simulink model "mrefrobotarm_previous_y_previous_u_previous_ref_cex"  (R2018b)
settings: Solver=FixedStepAuto  StartTime=0.0  StopTime=20  RelTol=1e-3  AbsTol=1e-6
undefined symbols (not defined in the file or in its folder): cc, options
libraries: neural x330, simulink x2
(part 9 of 13)

== system mrefrobotarm_previous_y_previous_u_previous_ref_cex/cex_m3/Layer 3/Delays 1 ==
  "p{3}" : Inport  PortDimensions=30
      mask Display: e = 0.06;c1 = [120 230 180]/255;c2 = ([120 230 180]+0)/(256+128);c3 = ([120 230 180]+128)/(256+128);patch([0 1 1 0],[0 0 1 1],c1);patch([0 1 1 1-e 1-e 0+e],[0 0 1 1-e 0+e 0+e],c2);patch([0 0 1 1-e 0+e 0+e],[0 1 1 1-e 1-e 0+e],c3);plot([0 1 1 0 0],[0 0 1 1 0]);
  mux : Mux  Inputs=1
      mask Display: e = 0.06;c1 = [120 150 230]/255;c2 = ([120 150 230]+0)/383;c3 = ([120 150 230]+128)/383;patch([0 1 1 0],[0 0 1 1],c1);patch([0 1 1 1-e 1-e 0+e],[0 0 1 1-e 0+e 0+e],c2);patch([0 0 1 1-e 0+e 0+e],[0 1 1 1-e 1-e 0+e],c3);plot([0 1 1 0 0],[0 0 1 1 0]);disp('Mux')
  "pd{3,2}" : Outport
      mask Display: e = 0.06;c1 = [120 230 180]/255;c2 = ([120 230 180]+0)/(256+128);c3 = ([120 230 180]+128)/(256+128);patch([0 1 1 0],[0 0 1 1],c1);patch([0 1 1 1-e 1-e 0+e],[0 0 1 1-e 0+e 0+e],c2);patch([0 0 1 1-e 0+e 0+e],[0 1 1 1-e 1-e 0+e],c3);plot([0 1 1 0 0],[0 0 1 1 0]);
  wires:
  "p{3}"/1 -> mux/1
  mux/1 -> "pd{3,2}"/1

== system mrefrobotarm_previous_y_previous_u_previous_ref_cex/cex_m3/Layer 3/LW{3,2} ==
  "ad{3,2}" : Inport  PortDimensions=30
      mask Display: e = 0.06;c1 = [120 230 180]/255;c2 = ([120 230 180]+0)/(256+128);c3 = ([120 230 180]+128)/(256+128);patch([0 1 1 0],[0 0 1 1],c1);patch([0 1 1 1-e 1-e 0+e],[0 0 1 1-e 0+e 0+e],c2);patch([0 0 1 1-e 0+e 0+e],[0 1 1 1-e 1-e 0+e],c3);plot([0 1 1 0 0],[0 0 1 1 0]);
  "IW{3,2}(1,:)'" : Constant  Value=[-0.4264094248819685351037378495675511658191680908203125;-0.391491550571647362044558349225553683936595916748046875;-0.207148976525499239897953884792514145374298095703125;0.438864475537191156551131143714883364737033843994140625;-0.253842970429255465614204467783565632998943328857421875;-0.310782373552643986780452678431174717843532562255859375;0.17090784249601165267762326038791798055171966552734375;0.48173109431363936305814377192291431128978729248046875;0.282586899793619117371434867891366593539714813232421875;0.01002122853356772480548642079156707040965557098388671875;-0.306381368505943496582943907924345694482326507568359375;0.099394743635973725748300466875662095844745635986328125;-0.320608327918287805413655178199405781924724578857421875;-0.250902128691253001324668048255261965095996856689453125;-0.080231422707110755521142664292710833251476287841796875;0.0929087546576900236150464706952334381639957427978515625;-0.1540763130365487565409665648985537700355052947998046875;0.280406867713617113935242741717956960201263427734375;-0.4379282806221624912978995780576951801776885986328125;0.304633634951007536972866773794521577656269073486328125;-0.09742255331069239743246868101778090931475162506103515625;-0.0928910076785210703231854267869493924081325531005859375;0.475898592804404330092182817679713480174541473388671875;0.0086807129518768309794918280886122374795377254486083984375;-0.479191188062265016611718237982131540775299072265625;0.2631734648013746014072467005462385714054107666015625;-0.010127174248898966613108285628186422400176525115966796875;-0.359889086073808706078835939479176886379718780517578125;-0.01097745989372158649521882267663386301137506961822509765625;-0.12277942593390335501712939958451897837221622467041015625]
      mask Display: e = 0.06;c1 = [120 150 230]/255;c2 = ([120 150 230]+0)/383;c3 = ([120 150 230]+128)/383;patch([0 1 1 0],[0 0 1 1],c1);patch([0 1 1 1-e 1-e 0+e],[0 0 1 1-e 0+e 0+e],c2);patch([0 0 1 1-e 0+e 0+e],[0 1 1 1-e 1-e 0+e],c3);plot([0 1 1 0 0],[0 0 1 1 0]);disp('weights');
  Mux : Mux  Inputs=1
      mask Display: e = 0.06;c1 = [120 150 230]/255;c2 = ([120 150 230]+0)/383;c3 = ([120 150 230]+128)/383;patch([0 1 1 0],[0 0 1 1],c1);patch([0 1 1 1-e 1-e 0+e],[0 0 1 1-e 0+e 0+e],c2);patch([0 0 1 1-e 0+e 0+e],[0 1 1 1-e 1-e 0+e],c3);plot([0 1 1 0 0],[0 0 1 1 0]);disp('Mux');
  dotprod1 : neural/Weight Functions/dotprod
  "lz{3,2}" : Outport
      mask Display: e = 0.06;c1 = [120 230 180]/255;c2 = ([120 230 180]+0)/(256+128);c3 = ([120 230 180]+128)/(256+128);patch([0 1 1 0],[0 0 1 1],c1);patch([0 1 1 1-e 1-e 0+e],[0 0 1 1-e 0+e 0+e],c2);patch([0 0 1 1-e 0+e 0+e],[0 1 1 1-e 1-e 0+e],c3);plot([0 1 1 0 0],[0 0 1 1 0]);
  wires:
  "IW{3,2}(1,:)'"/1 -> dotprod1/1
  "ad{3,2}"/1 -> dotprod1/2
  dotprod1/1 -> Mux/1
  Mux/1 -> "lz{3,2}"/1

== system mrefrobotarm_previous_y_previous_u_previous_ref_cex/cex_m4/Layer 1/Delays 1 ==
  "p{1}" : Inport  PortDimensions=10
      mask Display: e = 0.06;c1 = [120 230 180]/255;c2 = ([120 230 180]+0)/(256+128);c3 = ([120 230 180]+128)/(256+128);patch([0 1 1 0],[0 0 1 1],c1);patch([0 1 1 1-e 1-e 0+e],[0 0 1 1-e 0+e 0+e],c2);patch([0 0 1 1-e 0+e 0+e],[0 1 1 1-e 1-e 0+e],c3);plot([0 1 1 0 0],[0 0 1 1 0]);
  mux : Mux  Inputs=1
      mask Display: e = 0.06;c1 = [120 150 230]/255;c2 = ([120 150 230]+0)/383;c3 = ([120 150 230]+128)/383;patch([0 1 1 0],[0 0 1 1],c1);patch([0 1 1 1-e 1-e 0+e],[0 0 1 1-e 0+e 0+e],c2);patch([0 0 1 1-e 0+e 0+e],[0 1 1 1-e 1-e 0+e],c3);plot([0 1 1 0 0],[0 0 1 1 0]);disp('Mux')
  "pd{1,1}" : Outport
      mask Display: e = 0.06;c1 = [120 230 180]/255;c2 = ([120 230 180]+0)/(256+128);c3 = ([120 230 180]+128)/(256+128);patch([0 1 1 0],[0 0 1 1],c1);patch([0 1 1 1-e 1-e 0+e],[0 0 1 1-e 0+e 0+e],c2);patch([0 0 1 1-e 0+e 0+e],[0 1 1 1-e 1-e 0+e],c3);plot([0 1 1 0 0],[0 0 1 1 0]);
  wires:
  "p{1}"/1 -> mux/1
  mux/1 -> "pd{1,1}"/1

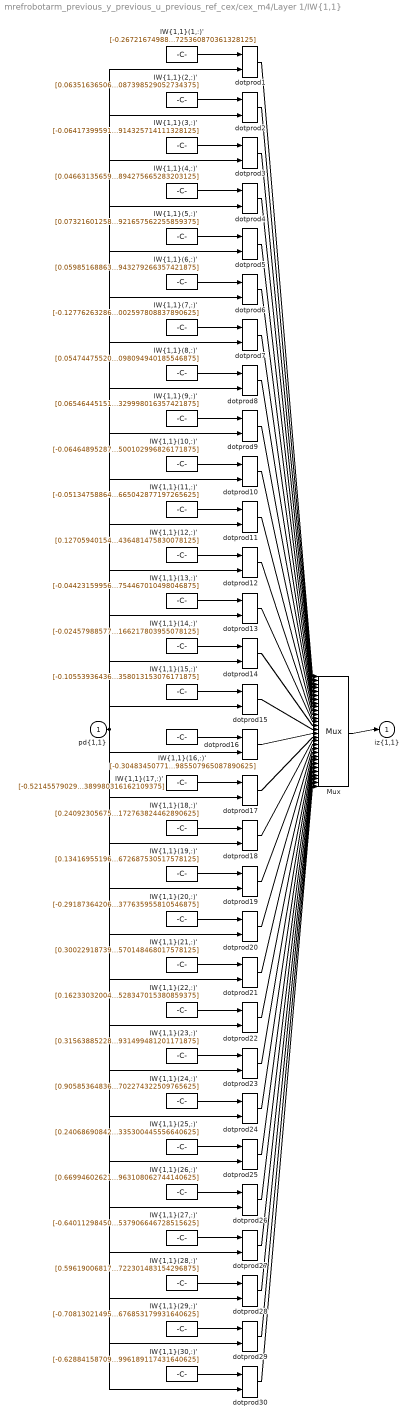
== system mrefrobotarm_previous_y_previous_u_previous_ref_cex/cex_m4/Layer 1/IW{1,1} ==
  "pd{1,1}" : Inport  PortDimensions=10
      mask Display: e = 0.06;c1 = [120 230 180]/255;c2 = ([120 230 180]+0)/(256+128);c3 = ([120 230 180]+128)/(256+128);patch([0 1 1 0],[0 0 1 1],c1);patch([0 1 1 1-e 1-e 0+e],[0 0 1 1-e 0+e 0+e],c2);patch([0 0 1 1-e 0+e 0+e],[0 1 1 1-e 1-e 0+e],c3);plot([0 1 1 0 0],[0 0 1 1 0]);
  "IW{1,1}(1,:)'" : Constant  Value=[-0.267216749881550141854091862114728428423404693603515625;-0.40822662087511296657993398184771649539470672607421875;-0.1379052433439487967969938608803204260766506195068359375;-0.10101957390506945133612504150733002461493015289306640625;-0.218242408285421018998562203705660067498683929443359375;-0.2333909870530341823524622668628580868244171142578125;-0.03607935037657590549020625303455744870007038116455078125;-0.204693462346923371608653496878105215728282928466796875;-0.0676737171591259289993303127630497328937053680419921875;-0.20060575168549832358877438309718854725360870361328125]
      mask Display: e = 0.06;c1 = [120 150 230]/255;c2 = ([120 150 230]+0)/383;c3 = ([120 150 230]+128)/383;patch([0 1 1 0],[0 0 1 1],c1);patch([0 1 1 1-e 1-e 0+e],[0 0 1 1-e 0+e 0+e],c2);patch([0 0 1 1-e 0+e 0+e],[0 1 1 1-e 1-e 0+e],c3);plot([0 1 1 0 0],[0 0 1 1 0]);disp('Weights');
  "IW{1,1}(10,:)'" : Constant  Value=[-0.06464895287319265271275270379192079417407512664794921875;0.0921228152977635883491558388413977809250354766845703125;0.0699758923557921852509622340221540071070194244384765625;0.039369719078938207601492393905573408119380474090576171875;0.2500761972795400023272804901353083550930023193359375;0.1424100538986860231549513855497934855520725250244140625;0.263550719297620916758972953175543807446956634521484375;0.178657006480026581130005070008337497711181640625;0.2561415896215992749063161681988276541233062744140625;-0.06333407118773848321069408484618179500102996826171875]
      mask Display: e = 0.06;c1 = [120 150 230]/255;c2 = ([120 150 230]+0)/383;c3 = ([120 150 230]+128)/383;patch([0 1 1 0],[0 0 1 1],c1);patch([0 1 1 1-e 1-e 0+e],[0 0 1 1-e 0+e 0+e],c2);patch([0 0 1 1-e 0+e 0+e],[0 1 1 1-e 1-e 0+e],c3);plot([0 1 1 0 0],[0 0 1 1 0]);disp('Weights');
  "IW{1,1}(11,:)'" : Constant  Value=[-0.051347588641863818603727764866562210954725742340087890625;0.261299948635366818816549994153319858014583587646484375;-0.07888061835908306840270398652137373574078083038330078125;-0.1396680730473503773136911831898032687604427337646484375;0.07888813015034022713134476134655415080487728118896484375;-0.03396823063257743691156775867057149298489093780517578125;-0.05818663428141730709075574168309685774147510528564453125;-0.207754130607128162377961189122288487851619720458984375;0.121149594677301630785137831480824388563632965087890625;-0.023398605256528072493527048436590121127665042877197265625]
      mask Display: e = 0.06;c1 = [120 150 230]/255;c2 = ([120 150 230]+0)/383;c3 = ([120 150 230]+128)/383;patch([0 1 1 0],[0 0 1 1],c1);patch([0 1 1 1-e 1-e 0+e],[0 0 1 1-e 0+e 0+e],c2);patch([0 0 1 1-e 0+e 0+e],[0 1 1 1-e 1-e 0+e],c3);plot([0 1 1 0 0],[0 0 1 1 0]);disp('Weights');
  "IW{1,1}(12,:)'" : Constant  Value=[0.1270594015435609069886169208984938450157642364501953125;-0.251472209491675646741981609011418186128139495849609375;0.00758860479230148536611277876318126800470054149627685546875;-0.07552348662196907425059322349625290371477603912353515625;-0.0189226418484879331527448442784589133225381374359130859375;-0.151454362118226548705735012845252640545368194580078125;0.006932621563510759678250483517558677704073488712310791015625;0.0379065119537769501523172266388428397476673126220703125;-0.12290012424222727938083465915042324922978878021240234375;0.115999064076067803785718979270313866436481475830078125]
      mask Display: e = 0.06;c1 = [120 150 230]/255;c2 = ([120 150 230]+0)/383;c3 = ([120 150 230]+128)/383;patch([0 1 1 0],[0 0 1 1],c1);patch([0 1 1 1-e 1-e 0+e],[0 0 1 1-e 0+e 0+e],c2);patch([0 0 1 1-e 0+e 0+e],[0 1 1 1-e 1-e 0+e],c3);plot([0 1 1 0 0],[0 0 1 1 0]);disp('Weights');
  "IW{1,1}(13,:)'" : Constant  Value=[-0.04423159956968956973977213920079520903527736663818359375;0.159509068566034528657837654463946819305419921875;-0.03746830256489484811677215247982530854642391204833984375;0.1024420286414695901999749594324384815990924835205078125;-0.1568938236393770668808400614580023102462291717529296875;-0.1263234848339660765237368877933477051556110382080078125;0.1373929609666244833210413389679160900413990020751953125;-0.07214503717479010813651285616288078017532825469970703125;0.0119749599667810895098352119703122298233211040496826171875;-0.07465610010787752937044814416367444209754467010498046875]
      mask Display: e = 0.06;c1 = [120 150 230]/255;c2 = ([120 150 230]+0)/383;c3 = ([120 150 230]+128)/383;patch([0 1 1 0],[0 0 1 1],c1);patch([0 1 1 1-e 1-e 0+e],[0 0 1 1-e 0+e 0+e],c2);patch([0 0 1 1-e 0+e 0+e],[0 1 1 1-e 1-e 0+e],c3);plot([0 1 1 0 0],[0 0 1 1 0]);disp('Weights');
  "IW{1,1}(14,:)'" : Constant  Value=[-0.0245798857762479124045018608057944220490753650665283203125;-0.10986830585016539585385686450536013580858707427978515625;-0.2240634718301251215866187749270466156303882598876953125;0.03927848130053805675299116728638182394206523895263671875;-0.1846276662278691083063364430927322246134281158447265625;0.0260786579550576179398202469883472076617181301116943359375;-0.0923985156179212285820767647237516939640045166015625;-0.060646538855653721322713778363322489894926548004150390625;-0.139029928035326488799938715601456351578235626220703125;0.02460306471988822629715087941804085858166217803955078125]
      mask Display: e = 0.06;c1 = [120 150 230]/255;c2 = ([120 150 230]+0)/383;c3 = ([120 150 230]+128)/383;patch([0 1 1 0],[0 0 1 1],c1);patch([0 1 1 1-e 1-e 0+e],[0 0 1 1-e 0+e 0+e],c2);patch([0 0 1 1-e 0+e 0+e],[0 1 1 1-e 1-e 0+e],c3);plot([0 1 1 0 0],[0 0 1 1 0]);disp('Weights');
  "IW{1,1}(15,:)'" : Constant  Value=[-0.105539364364973742294040448541636578738689422607421875;-0.0263920249190662502269955069778006873093545436859130859375;0.017234595038142376532963595536784850992262363433837890625;-0.255393520989991296143983845468028448522090911865234375;-0.035105650970056238857619490545403095893561840057373046875;-0.0163513867441485612197471510853574727661907672882080078125;-0.0295159521559936639800714175407847505994141101837158203125;-0.1673347691651354551822805660776793956756591796875;-0.037162506725512085836715669984187115915119647979736328125;0.005346155951647601871357107228277527610771358013153076171875]
      mask Display: e = 0.06;c1 = [120 150 230]/255;c2 = ([120 150 230]+0)/383;c3 = ([120 150 230]+128)/383;patch([0 1 1 0],[0 0 1 1],c1);patch([0 1 1 1-e 1-e 0+e],[0 0 1 1-e 0+e 0+e],c2);patch([0 0 1 1-e 0+e 0+e],[0 1 1 1-e 1-e 0+e],c3);plot([0 1 1 0 0],[0 0 1 1 0]);disp('Weights');
  "IW{1,1}(16,:)'" : Constant  Value=[-0.30483450771325137917955316879670135676860809326171875;0.056993584964788047975137175171767012216150760650634765625;-0.13938288150145983212979672316578216850757598876953125;-0.0225306251139089745716415080778460833244025707244873046875;0.01359296115692081551029612995762363425455987453460693359375;-0.1309181736384132654915646298832143656909465789794921875;0.09110308662115275402104686008897260762751102447509765625;-0.1684457458518295869254188801278360188007354736328125;-0.04626449882553897163806055914392345584928989410400390625;-0.284806204554836350784086107523762620985507965087890625]
      mask Display: e = 0.06;c1 = [120 150 230]/255;c2 = ([120 150 230]+0)/383;c3 = ([120 150 230]+128)/383;patch([0 1 1 0],[0 0 1 1],c1);patch([0 1 1 1-e 1-e 0+e],[0 0 1 1-e 0+e 0+e],c2);patch([0 0 1 1-e 0+e 0+e],[0 1 1 1-e 1-e 0+e],c3);plot([0 1 1 0 0],[0 0 1 1 0]);disp('Weights');
  "IW{1,1}(17,:)'" : Constant  Value=[-0.52145579029431754491952233365736901760101318359375;-0.324607409752539488589917482386226765811443328857421875;-0.0319440781114496974435468246156233362853527069091796875;-0.01239414051610091514754596886405124678276479244232177734375;-0.1914576463747985346497415548583376221358776092529296875;-0.157309606734231055558126399773755110800266265869140625;-0.32148224800624036756602208697586320340633392333984375;-0.284450749251240420090169891409459523856639862060546875;-0.1478505228260354187330705144631792791187763214111328125;-0.045385020230083082670713423567576683126389980316162109375]
      mask Display: e = 0.06;c1 = [120 150 230]/255;c2 = ([120 150 230]+0)/383;c3 = ([120 150 230]+128)/383;patch([0 1 1 0],[0 0 1 1],c1);patch([0 1 1 1-e 1-e 0+e],[0 0 1 1-e 0+e 0+e],c2);patch([0 0 1 1-e 0+e 0+e],[0 1 1 1-e 1-e 0+e],c3);plot([0 1 1 0 0],[0 0 1 1 0]);disp('Weights');
  "IW{1,1}(18,:)'" : Constant  Value=[0.2409230567548679424749735744626377709209918975830078125;0.49656984646448576459221158074797131121158599853515625;0.290985707265938586818521116583724506199359893798828125;0.352602910642589140177705075984704308211803436279296875;0.3085480397073692149234602766227908432483673095703125;0.222304352434349594691553875236422754824161529541015625;0.303863149672055243843971084061195142567157745361328125;0.0698155688711211419583690940271480940282344818115234375;-0.1600693098387457047326876136139617301523685455322265625;-0.429772611327940590175700208419584669172763824462890625]
      mask Display: e = 0.06;c1 = [120 150 230]/255;c2 = ([120 150 230]+0)/383;c3 = ([120 150 230]+128)/383;patch([0 1 1 0],[0 0 1 1],c1);patch([0 1 1 1-e 1-e 0+e],[0 0 1 1-e 0+e 0+e],c2);patch([0 0 1 1-e 0+e 0+e],[0 1 1 1-e 1-e 0+e],c3);plot([0 1 1 0 0],[0 0 1 1 0]);disp('Weights');
  "IW{1,1}(19,:)'" : Constant  Value=[0.1341695519644230116806937758155982010066509246826171875;-0.1742853076472074269620549102910445071756839752197265625;-0.03701738455975168984313228293103748001158237457275390625;0.076384486426226583244414314322057180106639862060546875;-0.01047937876791799928499759886335596092976629734039306640625;-0.12109423257529740303173326765318051911890506744384765625;0.0220112019456234764280821991633274592459201812744140625;-0.16146623763280143482035100532812066376209259033203125;0.06120155563627853456676319865437108092010021209716796875;-0.08720404259234344757079071541738812811672687530517578125]
      mask Display: e = 0.06;c1 = [120 150 230]/255;c2 = ([120 150 230]+0)/383;c3 = ([120 150 230]+128)/383;patch([0 1 1 0],[0 0 1 1],c1);patch([0 1 1 1-e 1-e 0+e],[0 0 1 1-e 0+e 0+e],c2);patch([0 0 1 1-e 0+e 0+e],[0 1 1 1-e 1-e 0+e],c3);plot([0 1 1 0 0],[0 0 1 1 0]);disp('Weights');
  "IW{1,1}(2,:)'" : Constant  Value=[0.06351636506590928321625000307903974317014217376708984375;0.11930786387308332796575172096709138713777065277099609375;0.1280645820977200644019688979824422858655452728271484375;0.162144232475708138796477442156174220144748687744140625;0.1871883600761256316591385484571219421923160552978515625;0.0168292633844707890944381034614707459695637226104736328125;0.1938829913256168435697901486491900868713855743408203125;0.06509252142771927707176615740536362864077091217041015625;-0.02851669131545607471789338660528301261365413665771484375;-0.318876840320537979778237058781087398529052734375]
      mask Display: e = 0.06;c1 = [120 150 230]/255;c2 = ([120 150 230]+0)/383;c3 = ([120 150 230]+128)/383;patch([0 1 1 0],[0 0 1 1],c1);patch([0 1 1 1-e 1-e 0+e],[0 0 1 1-e 0+e 0+e],c2);patch([0 0 1 1-e 0+e 0+e],[0 1 1 1-e 1-e 0+e],c3);plot([0 1 1 0 0],[0 0 1 1 0]);disp('Weights');
  "IW{1,1}(20,:)'" : Constant  Value=[-0.291873642062524918383559224821510724723339080810546875;0.0155193769184839742980575039155155536718666553497314453125;-0.25462870462001541138619131743325851857662200927734375;-0.046663558636088897646487794190761633217334747314453125;-0.2050390720883230877280567483467166312038898468017578125;-0.2490154875268562328916033266068552620708942413330078125;-0.273116089395899541703016666360781528055667877197265625;-0.289683676595492212157978428876958787441253662109375;-0.132150491808138259575144957125303335487842559814453125;-0.0552559521734092840006269398145377635955810546875]
      mask Display: e = 0.06;c1 = [120 150 230]/255;c2 = ([120 150 230]+0)/383;c3 = ([120 150 230]+128)/383;patch([0 1 1 0],[0 0 1 1],c1);patch([0 1 1 1-e 1-e 0+e],[0 0 1 1-e 0+e 0+e],c2);patch([0 0 1 1-e 0+e 0+e],[0 1 1 1-e 1-e 0+e],c3);plot([0 1 1 0 0],[0 0 1 1 0]);disp('Weights');
  "IW{1,1}(21,:)'" : Constant  Value=[0.300229187392162477632240324965096078813076019287109375;0.317431380612897717785614304375485517084598541259765625;0.11458850033386035194293839367674081586301326751708984375;0.176851946571799256702206548652611672878265380859375;0.07768512346275276148066524228852358646690845489501953125;0.178815523221328043224076509432052262127399444580078125;0.10338050103036089399921593212638981640338897705078125;0.018921033678644443021266141613523359410464763641357421875;0.189488271159305610158440913437516428530216217041015625;0.1903798222345019219847728209060733206570148468017578125]
      mask Display: e = 0.06;c1 = [120 150 230]/255;c2 = ([120 150 230]+0)/383;c3 = ([120 150 230]+128)/383;patch([0 1 1 0],[0 0 1 1],c1);patch([0 1 1 1-e 1-e 0+e],[0 0 1 1-e 0+e 0+e],c2);patch([0 0 1 1-e 0+e 0+e],[0 1 1 1-e 1-e 0+e],c3);plot([0 1 1 0 0],[0 0 1 1 0]);disp('Weights');
  "IW{1,1}(22,:)'" : Constant  Value=[0.162330320040409425974559098904137499630451202392578125;0.1760155520548265795088838103765738196671009063720703125;0.1980011245623203020027602860864135436713695526123046875;0.08825896072960770499804539213073439896106719970703125;0.214221740389516079883236443492933176457881927490234375;0.08709375089588149154717910960243898443877696990966796875;0.1432464034548406595082070680291508324444293975830078125;0.205133408044915255263873632429749704897403717041015625;0.1616554197014331284432131496942020021378993988037109375;0.1410755108505339361357755478820763528347015380859375]
      mask Display: e = 0.06;c1 = [120 150 230]/255;c2 = ([120 150 230]+0)/383;c3 = ([120 150 230]+128)/383;patch([0 1 1 0],[0 0 1 1],c1);patch([0 1 1 1-e 1-e 0+e],[0 0 1 1-e 0+e 0+e],c2);patch([0 0 1 1-e 0+e 0+e],[0 1 1 1-e 1-e 0+e],c3);plot([0 1 1 0 0],[0 0 1 1 0]);disp('Weights');
  "IW{1,1}(23,:)'" : Constant  Value=[0.3156388522827195952658030364545993506908416748046875;-0.0303480675321638748709318633700604550540447235107421875;0.0261651991707960406008393050569793558679521083831787109375;0.052469398667946427761155092639455688185989856719970703125;0.032880744367926283133751752529860823415219783782958984375;0.0942659029548157112454731532125151716172695159912109375;0.142636786970836426657882611834793351590633392333984375;-0.057596112250889619499361060661613009870052337646484375;0.0955492320642383763384941630647517740726470947265625;-0.07794382114178070863896863329500774852931499481201171875]
      mask Display: e = 0.06;c1 = [120 150 230]/255;c2 = ([120 150 230]+0)/383;c3 = ([120 150 230]+128)/383;patch([0 1 1 0],[0 0 1 1],c1);patch([0 1 1 1-e 1-e 0+e],[0 0 1 1-e 0+e 0+e],c2);patch([0 0 1 1-e 0+e 0+e],[0 1 1 1-e 1-e 0+e],c3);plot([0 1 1 0 0],[0 0 1 1 0]);disp('Weights');
  "IW{1,1}(24,:)'" : Constant  Value=[0.90585364836736703697539496715762652456760406494140625;-0.2426328840753690652132235072713228873908519744873046875;0.2290538535864212743575762942782603204250335693359375;0.0276980522269096758603001973142454517073929309844970703125;0.09685979922238562023206753792692325077950954437255859375;0.1261857423448861370562923411853262223303318023681640625;-0.09704113755403249996778214381265570409595966339111328125;0.1577690254322382801266400065287598408758640289306640625;0.025090152047807907920162762138716061599552631378173828125;0.10783235852078067174009134987500146962702274322509765625]
      mask Display: e = 0.06;c1 = [120 150 230]/255;c2 = ([120 150 230]+0)/383;c3 = ([120 150 230]+128)/383;patch([0 1 1 0],[0 0 1 1],c1);patch([0 1 1 1-e 1-e 0+e],[0 0 1 1-e 0+e 0+e],c2);patch([0 0 1 1-e 0+e 0+e],[0 1 1 1-e 1-e 0+e],c3);plot([0 1 1 0 0],[0 0 1 1 0]);disp('Weights');
  "IW{1,1}(25,:)'" : Constant  Value=[0.240686908421116674272610680418438278138637542724609375;-0.104028123549407769399266499021905474364757537841796875;-0.09450604313064690786827526380875497125089168548583984375;0.11409052644208968196881670564835076220333576202392578125;-0.069072497417360823046550422077416442334651947021484375;-0.1277032424560556045367576416538213379681110382080078125;0.060117468374489287097350853628086042590439319610595703125;0.087487371426137716667881250032223761081695556640625;-0.032553856975236307447207906307085067965090274810791015625;0.005567118611491368197763396352684139856137335300445556640625]
      mask Display: e = 0.06;c1 = [120 150 230]/255;c2 = ([120 150 230]+0)/383;c3 = ([120 150 230]+128)/383;patch([0 1 1 0],[0 0 1 1],c1);patch([0 1 1 1-e 1-e 0+e],[0 0 1 1-e 0+e 0+e],c2);patch([0 0 1 1-e 0+e 0+e],[0 1 1 1-e 1-e 0+e],c3);plot([0 1 1 0 0],[0 0 1 1 0]);disp('Weights');
  "IW{1,1}(26,:)'" : Constant  Value=[0.66994602621044474499711895987275056540966033935546875;0.2219850096971208441853917747721425257623195648193359375;0.176049719549269345630904126664972864091396331787109375;0.1226973401518094142215176134413923136889934539794921875;0.07370925043911900897963818124480894766747951507568359375;-0.07340785025997599577696206551991053856909275054931640625;0.042640181004205530979067617636246723122894763946533203125;-0.153863749044390318854169663609354756772518157958984375;-0.04609826544353955168897840621866635046899318695068359375;0.1366000115535325465376814690898754633963108062744140625]
      mask Display: e = 0.06;c1 = [120 150 230]/255;c2 = ([120 150 230]+0)/383;c3 = ([120 150 230]+128)/383;patch([0 1 1 0],[0 0 1 1],c1);patch([0 1 1 1-e 1-e 0+e],[0 0 1 1-e 0+e 0+e],c2);patch([0 0 1 1-e 0+e 0+e],[0 1 1 1-e 1-e 0+e],c3);plot([0 1 1 0 0],[0 0 1 1 0]);disp('Weights');
  "IW{1,1}(27,:)'" : Constant  Value=[-0.64011298450993125985775122899212874472141265869140625;0.1264277862932005336293883601683774031698703765869140625;-0.1885447022138225514620302192270173691213130950927734375;-0.09251043684248581866480520830009481869637966156005859375;0.103092036338989168076096802906249649822711944580078125;-0.00191654901815719908193813569852181899477727711200714111328125;-0.053867495492080121055611385827432968653738498687744140625;-0.039687340519823595397230775461139273829758167266845703125;-0.04914164559390850339770651089565944857895374298095703125;-0.0258128202979643374403995181864956975914537906646728515625]
      mask Display: e = 0.06;c1 = [120 150 230]/255;c2 = ([120 150 230]+0)/383;c3 = ([120 150 230]+128)/383;patch([0 1 1 0],[0 0 1 1],c1);patch([0 1 1 1-e 1-e 0+e],[0 0 1 1-e 0+e 0+e],c2);patch([0 0 1 1-e 0+e 0+e],[0 1 1 1-e 1-e 0+e],c3);plot([0 1 1 0 0],[0 0 1 1 0]);disp('Weights');
  "IW{1,1}(28,:)'" : Constant  Value=[0.5961900681766694187757593681453727185726165771484375;0.3430139714958020391577520058490335941314697265625;0.2341959314177390061306738289204076863825321197509765625;0.239631643975415087322033969030599109828472137451171875;0.1870724775690954799767240501751075498759746551513671875;0.1467603001405427820547089368119486607611179351806640625;0.10365323923488352353405872463554260320961475372314453125;0.1159775255986031095023491843676310963928699493408203125;0.05082354533000295326861106559590552933514118194580078125;-0.276042206131973333338436304984497837722301483154296875]
      mask Display: e = 0.06;c1 = [120 150 230]/255;c2 = ([120 150 230]+0)/383;c3 = ([120 150 230]+128)/383;patch([0 1 1 0],[0 0 1 1],c1);patch([0 1 1 1-e 1-e 0+e],[0 0 1 1-e 0+e 0+e],c2);patch([0 0 1 1-e 0+e 0+e],[0 1 1 1-e 1-e 0+e],c3);plot([0 1 1 0 0],[0 0 1 1 0]);disp('Weights');
  "IW{1,1}(29,:)'" : Constant  Value=[-0.70813021495672179295155501677072606980800628662109375;0.30675665628371129312057519200607202947139739990234375;-0.07076881114415210782819798396303667686879634857177734375;-0.0228481476932857925643549634742157650180160999298095703125;-0.082537316541165306471583562597515992820262908935546875;-0.0173445013735810428523453907700968557037413120269775390625;0.1688513365261939125350210133547079749405384063720703125;-0.07408557471998102050836365606301114894449710845947265625;-0.07749801166984006395299644509577774442732334136962890625;-0.18928142296034311531371940873214043676853179931640625]
      mask Display: e = 0.06;c1 = [120 150 230]/255;c2 = ([120 150 230]+0)/383;c3 = ([120 150 230]+128)/383;patch([0 1 1 0],[0 0 1 1],c1);patch([0 1 1 1-e 1-e 0+e],[0 0 1 1-e 0+e 0+e],c2);patch([0 0 1 1-e 0+e 0+e],[0 1 1 1-e 1-e 0+e],c3);plot([0 1 1 0 0],[0 0 1 1 0]);disp('Weights');
  "IW{1,1}(3,:)'" : Constant  Value=[-0.064173995914235393289715148057439364492893218994140625;-0.0059172667376275987771716557972467853687703609466552734375;0.05749714985246447140898595762337208725512027740478515625;-0.0899378683654476207554040456670918501913547515869140625;0.078819850763461707376933418345288373529911041259765625;0.0253495636063069233745448372019382077269256114959716796875;-0.0182511162189372307118606642006852780468761920928955078125;-0.0924131757659971686535982371424324810504913330078125;0.0010697191710963248334476105583235039375722408294677734375;0.1566136603183161668528811105716158635914325714111328125]
      mask Display: e = 0.06;c1 = [120 150 230]/255;c2 = ([120 150 230]+0)/383;c3 = ([120 150 230]+128)/383;patch([0 1 1 0],[0 0 1 1],c1);patch([0 1 1 1-e 1-e 0+e],[0 0 1 1-e 0+e 0+e],c2);patch([0 0 1 1-e 0+e 0+e],[0 1 1 1-e 1-e 0+e],c3);plot([0 1 1 0 0],[0 0 1 1 0]);disp('Weights');
  "IW{1,1}(30,:)'" : Constant  Value=[-0.628841587095009924013311319868080317974090576171875;0.1088899533473890179902099362152512185275554656982421875;-0.06463334913051617391932524014919181354343891143798828125;-0.043920919679465507401427970535223721526563167572021484375;-0.09722145811493441980299934357390156947076320648193359375;-0.051994330993742461644036012557990034110844135284423828125;0.1151241109324362132948493808726198039948940277099609375;0.0271505797353484117084843063594234990887343883514404296875;-0.0624483511445974859288554625891265459358692169189453125;-0.2341109402932441130307239518515416420996189117431640625]
      mask Display: e = 0.06;c1 = [120 150 230]/255;c2 = ([120 150 230]+0)/383;c3 = ([120 150 230]+128)/383;patch([0 1 1 0],[0 0 1 1],c1);patch([0 1 1 1-e 1-e 0+e],[0 0 1 1-e 0+e 0+e],c2);patch([0 0 1 1-e 0+e 0+e],[0 1 1 1-e 1-e 0+e],c3);plot([0 1 1 0 0],[0 0 1 1 0]);disp('Weights');
  "IW{1,1}(4,:)'" : Constant  Value=[0.0466313565929649398444922780981869436800479888916015625;-0.06226913105247489088611700935871340334415435791015625;-0.01544836403327122346940125652281494694761931896209716796875;0.03466835985496351246748503172057098709046840667724609375;0.07173125569554179847830965854882379062473773956298828125;0.153078658361084196659618328340002335608005523681640625;0.0770878264398895118869603493294562213122844696044921875;0.1874709283106799073692627644049935042858123779296875;0.08115331332375307071824721560915349982678890228271484375;0.0909525515275941831561112849158234894275665283203125]
      mask Display: e = 0.06;c1 = [120 150 230]/255;c2 = ([120 150 230]+0)/383;c3 = ([120 150 230]+128)/383;patch([0 1 1 0],[0 0 1 1],c1);patch([0 1 1 1-e 1-e 0+e],[0 0 1 1-e 0+e 0+e],c2);patch([0 0 1 1-e 0+e 0+e],[0 1 1 1-e 1-e 0+e],c3);plot([0 1 1 0 0],[0 0 1 1 0]);disp('Weights');
  "IW{1,1}(5,:)'" : Constant  Value=[0.07321601258536401812815341827445081435143947601318359375;-0.22569618673739311187631528810015879571437835693359375;0.1376235218885525635190703042098903097212314605712890625;0.0947860079499896757138088787542073987424373626708984375;0.1290056428927640330694970316471881233155727386474609375;0.053390939220054646485724703097730525769293308258056640625;-0.045191743751136388695943679749689181335270404815673828125;0.056231567537908866416529463094775564968585968017578125;-0.2466164700931786357696040568043827079236507415771484375;-0.20638216121557417803700218428275547921657562255859375]
      mask Display: e = 0.06;c1 = [120 150 230]/255;c2 = ([120 150 230]+0)/383;c3 = ([120 150 230]+128)/383;patch([0 1 1 0],[0 0 1 1],c1);patch([0 1 1 1-e 1-e 0+e],[0 0 1 1-e 0+e 0+e],c2);patch([0 0 1 1-e 0+e 0+e],[0 1 1 1-e 1-e 0+e],c3);plot([0 1 1 0 0],[0 0 1 1 0]);disp('Weights');
  "IW{1,1}(6,:)'" : Constant  Value=[0.05985168863605760947166345431469380855560302734375;-0.002159573538259234627700866582244998426176607608795166015625;-0.11318048141550020313506053071250789798796176910400390625;0.045337237095633316219522868095737067051231861114501953125;0.144154365313161336725755745646893046796321868896484375;0.06093673556748956110507009498178376816213130950927734375;-0.060293185465568922831725018340875976718962192535400390625;0.0227417706844570514934655847127942251972854137420654296875;-0.07437535283304806676962783740236773155629634857177734375;0.126522101641080630951563534836168400943279266357421875]
      mask Display: e = 0.06;c1 = [120 150 230]/255;c2 = ([120 150 230]+0)/383;c3 = ([120 150 230]+128)/383;patch([0 1 1 0],[0 0 1 1],c1);patch([0 1 1 1-e 1-e 0+e],[0 0 1 1-e 0+e 0+e],c2);patch([0 0 1 1-e 0+e 0+e],[0 1 1 1-e 1-e 0+e],c3);plot([0 1 1 0 0],[0 0 1 1 0]);disp('Weights');
  "IW{1,1}(7,:)'" : Constant  Value=[-0.1277626328603604921596570420661009848117828369140625;-0.46443151291336259856024071268620900809764862060546875;0.044606677753775601791286220532128936611115932464599609375;-0.136410331273810248031708169946796260774135589599609375;-0.0770422591237390486096359154544188641011714935302734375;-0.051187319207494509643030511369943269528448581695556640625;-0.09003239138660514007117541268598870374262332916259765625;-0.005325811764632123850027323186395733500830829143524169921875;-0.02833124307385037621287438014405779540538787841796875;0.198670566199726617018228580491268076002597808837890625]
      mask Display: e = 0.06;c1 = [120 150 230]/255;c2 = ([120 150 230]+0)/383;c3 = ([120 150 230]+128)/383;patch([0 1 1 0],[0 0 1 1],c1);patch([0 1 1 1-e 1-e 0+e],[0 0 1 1-e 0+e 0+e],c2);patch([0 0 1 1-e 0+e 0+e],[0 1 1 1-e 1-e 0+e],c3);plot([0 1 1 0 0],[0 0 1 1 0]);disp('Weights');
  "IW{1,1}(8,:)'" : Constant  Value=[0.054744755203041874092040330879171960987150669097900390625;-0.001305994968348087904852494745000512921251356601715087890625;-0.09307953323685579094526332255554734729230403900146484375;-0.08109344435434541475959946410512202419340610504150390625;-0.0907065859835935739408085964896599762141704559326171875;-0.0220450076101698366759507052847766317427158355712890625;-0.026212681759366772415997814960064715705811977386474609375;0.1228943021643547073296076632686890661716461181640625;0.08801937892250617789802191737180692143738269805908203125;0.08659338115619912012999037642657640390098094940185546875]
      mask Display: e = 0.06;c1 = [120 150 230]/255;c2 = ([120 150 230]+0)/383;c3 = ([120 150 230]+128)/383;patch([0 1 1 0],[0 0 1 1],c1);patch([0 1 1 1-e 1-e 0+e],[0 0 1 1-e 0+e 0+e],c2);patch([0 0 1 1-e 0+e 0+e],[0 1 1 1-e 1-e 0+e],c3);plot([0 1 1 0 0],[0 0 1 1 0]);disp('Weights');
  "IW{1,1}(9,:)'" : Constant  Value=[0.06546445151039102794410240448996773920953273773193359375;0.38763234071624308452186369322589598596096038818359375;-0.00672576750667506530201311676364639424718916416168212890625;0.110151702288806163654300007692654617130756378173828125;0.1013987501450804573632780147818266414105892181396484375;0.051810761808782891668645476102028624154627323150634765625;0.0494189364730958924365467055395129136741161346435546875;-0.026199443819789280940568687583436258137226104736328125;-0.0025078487207655822226193276236472229356877505779266357421875;-0.279777179941980147503954867715947329998016357421875]
      mask Display: e = 0.06;c1 = [120 150 230]/255;c2 = ([120 150 230]+0)/383;c3 = ([120 150 230]+128)/383;patch([0 1 1 0],[0 0 1 1],c1);patch([0 1 1 1-e 1-e 0+e],[0 0 1 1-e 0+e 0+e],c2);patch([0 0 1 1-e 0+e 0+e],[0 1 1 1-e 1-e 0+e],c3);plot([0 1 1 0 0],[0 0 1 1 0]);disp('Weights');
  Mux : Mux  Inputs=30
      mask Display: e = 0.06;c1 = [120 150 230]/255;c2 = ([120 150 230]+0)/383;c3 = ([120 150 230]+128)/383;patch([0 1 1 0],[0 0 1 1],c1);patch([0 1 1 1-e 1-e 0+e],[0 0 1 1-e 0+e 0+e],c2);patch([0 0 1 1-e 0+e 0+e],[0 1 1 1-e 1-e 0+e],c3);plot([0 1 1 0 0],[0 0 1 1 0]);disp('Mux');
  dotprod{1..30} (30 alike) : neural/Weight Functions/dotprod
  "iz{1,1}" : Outport
      mask Display: e = 0.06;c1 = [120 230 180]/255;c2 = ([120 230 180]+0)/(256+128);c3 = ([120 230 180]+128)/(256+128);patch([0 1 1 0],[0 0 1 1],c1);patch([0 1 1 1-e 1-e 0+e],[0 0 1 1-e 0+e 0+e],c2);patch([0 0 1 1-e 0+e 0+e],[0 1 1 1-e 1-e 0+e],c3);plot([0 1 1 0 0],[0 0 1 1 0]);
  wires:
  "IW{1,1}(1,:)'"/1 -> dotprod1/1
  "pd{1,1}"/1 -> dotprod1/2, dotprod2/2, dotprod3/2, dotprod4/2, dotprod5/2, dotprod6/2, dotprod7/2, dotprod8/2, dotprod9/2, dotprod10/2, dotprod11/2, dotprod12/2, dotprod13/2, dotprod14/2, dotprod15/2, dotprod16/2, dotprod17/2, dotprod18/2, dotprod19/2, dotprod20/2, dotprod21/2, dotprod22/2, dotprod23/2, dotprod24/2, dotprod25/2, dotprod26/2, dotprod27/2, dotprod28/2, dotprod29/2, dotprod30/2
  dotprod1/1 -> Mux/1
  "IW{1,1}(2,:)'"/1 -> dotprod2/1
  dotprod2/1 -> Mux/2
  "IW{1,1}(3,:)'"/1 -> dotprod3/1
  dotprod3/1 -> Mux/3
  "IW{1,1}(4,:)'"/1 -> dotprod4/1
  dotprod4/1 -> Mux/4
  "IW{1,1}(5,:)'"/1 -> dotprod5/1
  dotprod5/1 -> Mux/5
  "IW{1,1}(6,:)'"/1 -> dotprod6/1
  dotprod6/1 -> Mux/6
  "IW{1,1}(7,:)'"/1 -> dotprod7/1
  dotprod7/1 -> Mux/7
  "IW{1,1}(8,:)'"/1 -> dotprod8/1
  dotprod8/1 -> Mux/8
  "IW{1,1}(9,:)'"/1 -> dotprod9/1
  dotprod9/1 -> Mux/9
  "IW{1,1}(10,:)'"/1 -> dotprod10/1
  dotprod10/1 -> Mux/10
  "IW{1,1}(11,:)'"/1 -> dotprod11/1
  dotprod11/1 -> Mux/11
  "IW{1,1}(12,:)'"/1 -> dotprod12/1
  dotprod12/1 -> Mux/12
  "IW{1,1}(13,:)'"/1 -> dotprod13/1
  dotprod13/1 -> Mux/13
  "IW{1,1}(14,:)'"/1 -> dotprod14/1
  dotprod14/1 -> Mux/14
  "IW{1,1}(15,:)'"/1 -> dotprod15/1
  dotprod15/1 -> Mux/15
  "IW{1,1}(16,:)'"/1 -> dotprod16/1
  dotprod16/1 -> Mux/16
  "IW{1,1}(17,:)'"/1 -> dotprod17/1
  dotprod17/1 -> Mux/17
  "IW{1,1}(18,:)'"/1 -> dotprod18/1
  dotprod18/1 -> Mux/18
  "IW{1,1}(19,:)'"/1 -> dotprod19/1
  dotprod19/1 -> Mux/19
  "IW{1,1}(20,:)'"/1 -> dotprod20/1
  dotprod20/1 -> Mux/20
  "IW{1,1}(21,:)'"/1 -> dotprod21/1
  dotprod21/1 -> Mux/21
  "IW{1,1}(22,:)'"/1 -> dotprod22/1
  dotprod22/1 -> Mux/22
  "IW{1,1}(23,:)'"/1 -> dotprod23/1
  dotprod23/1 -> Mux/23
  "IW{1,1}(24,:)'"/1 -> dotprod24/1
  dotprod24/1 -> Mux/24
  "IW{1,1}(25,:)'"/1 -> dotprod25/1
  dotprod25/1 -> Mux/25
  "IW{1,1}(26,:)'"/1 -> dotprod26/1
  dotprod26/1 -> Mux/26
  "IW{1,1}(27,:)'"/1 -> dotprod27/1
  dotprod27/1 -> Mux/27
  "IW{1,1}(28,:)'"/1 -> dotprod28/1
  dotprod28/1 -> Mux/28
  "IW{1,1}(29,:)'"/1 -> dotprod29/1
  dotprod29/1 -> Mux/29
  "IW{1,1}(30,:)'"/1 -> dotprod30/1
  dotprod30/1 -> Mux/30
  Mux/1 -> "iz{1,1}"/1

== system mrefrobotarm_previous_y_previous_u_previous_ref_cex/cex_m4/Layer 2/Delays 1 ==
  "p{2}" : Inport  PortDimensions=30
      mask Display: e = 0.06;c1 = [120 230 180]/255;c2 = ([120 230 180]+0)/(256+128);c3 = ([120 230 180]+128)/(256+128);patch([0 1 1 0],[0 0 1 1],c1);patch([0 1 1 1-e 1-e 0+e],[0 0 1 1-e 0+e 0+e],c2);patch([0 0 1 1-e 0+e 0+e],[0 1 1 1-e 1-e 0+e],c3);plot([0 1 1 0 0],[0 0 1 1 0]);
  mux : Mux  Inputs=1
      mask Display: e = 0.06;c1 = [120 150 230]/255;c2 = ([120 150 230]+0)/383;c3 = ([120 150 230]+128)/383;patch([0 1 1 0],[0 0 1 1],c1);patch([0 1 1 1-e 1-e 0+e],[0 0 1 1-e 0+e 0+e],c2);patch([0 0 1 1-e 0+e 0+e],[0 1 1 1-e 1-e 0+e],c3);plot([0 1 1 0 0],[0 0 1 1 0]);disp('Mux')
  "pd{2,1}" : Outport
      mask Display: e = 0.06;c1 = [120 230 180]/255;c2 = ([120 230 180]+0)/(256+128);c3 = ([120 230 180]+128)/(256+128);patch([0 1 1 0],[0 0 1 1],c1);patch([0 1 1 1-e 1-e 0+e],[0 0 1 1-e 0+e 0+e],c2);patch([0 0 1 1-e 0+e 0+e],[0 1 1 1-e 1-e 0+e],c3);plot([0 1 1 0 0],[0 0 1 1 0]);
  wires:
  "p{2}"/1 -> mux/1
  mux/1 -> "pd{2,1}"/1
